simulink library "tqr"  (R2021b)
settings: Solver=VariableStepAuto  StartTime=0.0  StopTime=10.0  RelTol=1e-3
undefined symbols (not defined in the file or in its folder): ATQR_AltRDCActiveREDUInc_X_pct, ATQR_AltRDCActiveREDUInc_Y_enum, ATQR_AltRDCActiveREDUTs_X_pct, ATQR_AltRDCActiveREDUTs_Y_enum, ATQR_CreepREDUTqIncSR_X_rpm, ATQR_CreepREDUTqIncSR_Y_Nm, ATQR_CreepREDUTs_X_rpm, ATQR_CreepREDUTs_Y_Nm, ATQR_EcoTqRrIncGain_X_Nm, ATQR_EcoTqRrIncGain_Y_pct, ATQR_EL1REDUTqDecSR_Y_Nm, ATQR_EL1REDUTqIncSR_X_rpm, ATQR_EL1REDUTqIncSR_Y_pct, ATQR_EL1REDUTs_X_rpm, ATQR_EL1REDUTs_Y_Nm, ATQR_NL1REDUTqDecSR_Y_Nm, ATQR_NL1REDUTqIncSR_X_rpm, ATQR_NL1REDUTqIncSR_Y_pct, ATQR_NL1REDUTs_X_rpm, ATQR_NL1REDUTs_Y_Nm, ATQR_NormalTqRrIncGain_X_Nm, ATQR_NormalTqRrIncGain_Y_pct, ATQR_REDUTIPOutTs_X_rpm, ATQR_RrNegRateLimitIncN_X_rpm, ATQR_RrNegRateLimitIncN_Y_Nm, ATQR_RrPosRateLimitIncN_X_rpm, ATQR_RrPosRateLimitIncN_Y_Nm, ATQR_RTqZeroTransUpBoundN_X_rpm, ATQR_SL1REDUTqDecSR_Y_Nm, ATQR_SL1REDUTqIncSR_X_rpm, ATQR_SL1REDUTqIncSR_Y_pct, ATQR_SL1REDUTs_X_rpm, ATQR_SL1REDUTs_Y_Nm, ATQR_SportTqRrIncGain_X_Nm, ATQR_SportTqRrIncGain_Y_pct, ENUM_CANRDCACTSTA_EXITIMMEDIATELY, ENUM_DRIVEMODE_ECO, ENUM_DRIVEMODE_NRM, ENUM_DRIVEMODE_SPORT, ENUM_GEARACTUALPOSN_R, ENUM_RDCACTSTA_NOREQUEST, ENUM_TQZEROTRANS_NEGATIVE, ENUM_TQZEROTRANS_NOZEROTRANS, ENUM_TQZEROTRANS_POSITIVE, FALSE, KTQD_FrTMTotalGearRatio_gain, KTQD_RrTMTotalGearRatio_gain, KTQR_ARegenLatchEnTq_Nm, KTQR_DriveModeChangeTq_Nm, KTQR_DriveModeCMDTqDev_Nm, KTQR_FinalFEDUTrqLowLim_Nm, KTQR_FinalFEDUTrqUpLim_Nm, KTQR_FinalREDUTrqLowLim_Nm, KTQR_FinalREDUTrqUpLim_Nm, KTQR_FrTMGearEff_c, KTQR_GearEnChangeTq_Nm, KTQR_PreLoadTs_c, KTQR_RrTMGearEff_c, KTQR_TIPOutTsAPS_pct, KTQR_TIPOutTsSpd_kph ... (+44)
libraries: hcu_lib x7, simulink x6
(part 3 of 3)

== system tqr/TQR/Determine Torque Request/TorqueArbitrament/TorqueSmooth/Rear wheel rate limit determination/VTQR_SPORTREDURateLimitInc_Nm ==
  VDHP_ActAPSPosn_pct : Inport
  VTQD_TqTargetShaftSpd_rpm : Inport  Port=2
  VTQD_RegenMode_enum : Inport  Port=3
  VTQR_REDUWhlTqReqSmoothDelay_Nm : Inport  Port=4
  Action Port : ActionPort
  MTQR_SL1REDUTqIncSR_Z_Nm : Lookup_n-D  BreakpointsForDimension1=ATQR_SL1REDUTqIncSR_Y_pct  BreakpointsForDimension2=ATQR_SL1REDUTqIncSR_X_rpm  Table=MTQR_SL1REDUTqIncSR_Z_Nm  ExtrapMethod=Clip  InternalRulePriority=Speed  RndMeth=Simplest  InputSameDT=on
      settings: InputPortMap=u0,u1
  MTQR_SportTqRrIncGain_Z_c : Lookup_n-D  BreakpointsForDimension1=ATQR_SportTqRrIncGain_Y_pct  BreakpointsForDimension2=ATQR_SportTqRrIncGain_X_Nm  Table=MTQR_SportTqRrIncGain_Z_c  ExtrapMethod=Clip  InternalRulePriority=Speed  RndMeth=Simplest  InputSameDT=on
      settings: InputPortMap=u0,u1
  Product : Product
  Terminator : Terminator
  VTQR_SPORTREDURateLimitInc_Nm : Outport
  wires:
  VDHP_ActAPSPosn_pct/1 -> [VDHP_ActAPSPosn_pct]
  VTQD_TqTargetShaftSpd_rpm/1 -> [VTQD_TqTargetShaftSpd_rpm]
  VTQD_RegenMode_enum/1 -> Terminator/1
  [VTQR_REDUWhlTqReqSmoothDelay_Nm] -> MTQR_SportTqRrIncGain_Z_c/2
  [VDHP_ActAPSPosn_pct] -> MTQR_SportTqRrIncGain_Z_c/1
  VTQR_REDUWhlTqReqSmoothDelay_Nm/1 -> [VTQR_REDUWhlTqReqSmoothDelay_Nm]
  MTQR_SportTqRrIncGain_Z_c/1 -> [VTQR_SportTqRrIncGain_c]  "VTQR_SportTqRrIncGain_c"
  MTQR_SL1REDUTqIncSR_Z_Nm/1 -> Product/1
  Product/1 -> VTQR_SPORTREDURateLimitInc_Nm/1  "VTQR_SPORTREDURateLimitInc_Nm"
  [VDHP_ActAPSPosn_pct] -> MTQR_SL1REDUTqIncSR_Z_Nm/1
  [VTQD_TqTargetShaftSpd_rpm] -> MTQR_SL1REDUTqIncSR_Z_Nm/2
  [VTQR_SportTqRrIncGain_c] -> Product/2

== system tqr/TQR/Determine Torque Request/TorqueArbitrament/TorqueSmooth/Rear wheel rate limit determination/Negative Rate limit Determination/VTQR_RrNegRateLimitDecE_Nm ==
  VTQD_TqTargetShaftSpd_rpm : Inport
  VTQR_REDUWhlTqReqSmoothDelay_Nm : Inport  Port=2
  Action Port : ActionPort
  MTQR_RrNegRateLimitDecE_Z_Nm : Lookup_n-D  BreakpointsForDimension1=ATQR_RrNegRateLimitIncN_Y_Nm  BreakpointsForDimension2=ATQR_RrNegRateLimitIncN_X_rpm  Table=MTQR_RrNegRateLimitDecE_Z_Nm  ExtrapMethod=Clip  UseLastTableValue=on  InternalRulePriority=Speed  RndMeth=Simplest  InputSameDT=on
      settings: InputPortMap=u0,u1
  VTQR_RrNegRateLimitDecE_Nm : Outport
  wires:
  MTQR_RrNegRateLimitDecE_Z_Nm/1 -> VTQR_RrNegRateLimitDecE_Nm/1  "VTQR_RrNegRateLimitDecE_Nm"
  VTQR_REDUWhlTqReqSmoothDelay_Nm/1 -> MTQR_RrNegRateLimitDecE_Z_Nm/1
  VTQD_TqTargetShaftSpd_rpm/1 -> MTQR_RrNegRateLimitDecE_Z_Nm/2

== system tqr/TQR/Determine Torque Request/TorqueArbitrament/TorqueSmooth/Rear wheel rate limit determination/Negative Rate limit Determination/VTQR_RrNegRateLimitDecN_Nm ==
  VTQD_TqTargetShaftSpd_rpm : Inport
  VTQR_REDUWhlTqReqSmoothDelay_Nm : Inport  Port=2
  Action Port : ActionPort
  MTQR_RrNegRateLimitDecN_Z_Nm : Lookup_n-D  BreakpointsForDimension1=ATQR_RrNegRateLimitIncN_Y_Nm  BreakpointsForDimension2=ATQR_RrNegRateLimitIncN_X_rpm  Table=MTQR_RrNegRateLimitDecN_Z_Nm  ExtrapMethod=Clip  UseLastTableValue=on  InternalRulePriority=Speed  RndMeth=Simplest  InputSameDT=on
      settings: InputPortMap=u0,u1
  VTQR_RrNegRateLimitDecN_Nm : Outport
  wires:
  MTQR_RrNegRateLimitDecN_Z_Nm/1 -> VTQR_RrNegRateLimitDecN_Nm/1  "VTQR_RrNegRateLimitDecN_Nm"
  VTQR_REDUWhlTqReqSmoothDelay_Nm/1 -> MTQR_RrNegRateLimitDecN_Z_Nm/1
  VTQD_TqTargetShaftSpd_rpm/1 -> MTQR_RrNegRateLimitDecN_Z_Nm/2

== system tqr/TQR/Determine Torque Request/TorqueArbitrament/TorqueSmooth/Rear wheel rate limit determination/Negative Rate limit Determination/VTQR_RrNegRateLimitDecS_Nm ==
  VTQD_TqTargetShaftSpd_rpm : Inport
  VTQR_REDUWhlTqReqSmoothDelay_Nm : Inport  Port=2
  Action Port : ActionPort
  MTQR_RrNegRateLimitDecE_Z_Nm : Lookup_n-D  BreakpointsForDimension1=ATQR_RrNegRateLimitIncN_Y_Nm  BreakpointsForDimension2=ATQR_RrNegRateLimitIncN_X_rpm  Table=MTQR_RrNegRateLimitDecS_Z_Nm  ExtrapMethod=Clip  UseLastTableValue=on  InternalRulePriority=Speed  RndMeth=Simplest  InputSameDT=on
      settings: InputPortMap=u0,u1
  VTQR_RrNegRateLimitDecS_Nm : Outport
  wires:
  MTQR_RrNegRateLimitDecE_Z_Nm/1 -> VTQR_RrNegRateLimitDecS_Nm/1  "VTQR_RrNegRateLimitDecS_Nm"
  VTQD_TqTargetShaftSpd_rpm/1 -> MTQR_RrNegRateLimitDecE_Z_Nm/2
  VTQR_REDUWhlTqReqSmoothDelay_Nm/1 -> MTQR_RrNegRateLimitDecE_Z_Nm/1

== system tqr/TQR/Determine Torque Request/TorqueArbitrament/TorqueSmooth/Rear wheel rate limit determination/Negative Rate limit Determination/VTQR_RrNegRateLimitIncE_Nm ==
  VTQD_TqTargetShaftSpd_rpm : Inport
  VTQR_REDUWhlTqReqSmoothDelay_Nm : Inport  Port=2
  Action Port : ActionPort
  MTQR_RrNegRateLimitIncE_Z_Nm : Lookup_n-D  BreakpointsForDimension1=ATQR_RrNegRateLimitIncN_Y_Nm  BreakpointsForDimension2=ATQR_RrNegRateLimitIncN_X_rpm  Table=MTQR_RrNegRateLimitIncE_Z_Nm  ExtrapMethod=Clip  UseLastTableValue=on  InternalRulePriority=Speed  RndMeth=Simplest  InputSameDT=on
      settings: InputPortMap=u0,u1
  VTQR_RrNegRateLimitIncE_Nm : Outport
  wires:
  MTQR_RrNegRateLimitIncE_Z_Nm/1 -> VTQR_RrNegRateLimitIncE_Nm/1  "VTQR_RrNegRateLimitIncE_Nm"
  VTQR_REDUWhlTqReqSmoothDelay_Nm/1 -> MTQR_RrNegRateLimitIncE_Z_Nm/1
  VTQD_TqTargetShaftSpd_rpm/1 -> MTQR_RrNegRateLimitIncE_Z_Nm/2

== system tqr/TQR/Determine Torque Request/TorqueArbitrament/TorqueSmooth/Rear wheel rate limit determination/Negative Rate limit Determination/VTQR_RrNegRateLimitIncN_Nm ==
  VTQD_TqTargetShaftSpd_rpm : Inport
  VTQR_REDUWhlTqReqSmoothDelay_Nm : Inport  Port=2
  Action Port : ActionPort
  MTQR_RrNegRateLimitIncN_Z_Nm : Lookup_n-D  BreakpointsForDimension1=ATQR_RrNegRateLimitIncN_Y_Nm  BreakpointsForDimension2=ATQR_RrNegRateLimitIncN_X_rpm  Table=MTQR_RrNegRateLimitIncN_Z_Nm  ExtrapMethod=Clip  UseLastTableValue=on  InternalRulePriority=Speed  RndMeth=Simplest  InputSameDT=on
      settings: InputPortMap=u0,u1
  VTQR_RrNegRateLimitIncN_Nm : Outport
  wires:
  MTQR_RrNegRateLimitIncN_Z_Nm/1 -> VTQR_RrNegRateLimitIncN_Nm/1  "VTQR_RrNegRateLimitIncN_Nm"
  VTQR_REDUWhlTqReqSmoothDelay_Nm/1 -> MTQR_RrNegRateLimitIncN_Z_Nm/1
  VTQD_TqTargetShaftSpd_rpm/1 -> MTQR_RrNegRateLimitIncN_Z_Nm/2

== system tqr/TQR/Determine Torque Request/TorqueArbitrament/TorqueSmooth/Rear wheel rate limit determination/Negative Rate limit Determination/VTQR_RrNegRateLimitIncS_Nm ==
  VTQD_TqTargetShaftSpd_rpm : Inport
  VTQR_REDUWhlTqReqSmoothDelay_Nm : Inport  Port=2
  Action Port : ActionPort
  MTQR_RrNegRateLimitIncS_Z_Nm : Lookup_n-D  BreakpointsForDimension1=ATQR_RrNegRateLimitIncN_Y_Nm  BreakpointsForDimension2=ATQR_RrNegRateLimitIncN_X_rpm  Table=MTQR_RrNegRateLimitIncS_Z_Nm  ExtrapMethod=Clip  UseLastTableValue=on  InternalRulePriority=Speed  RndMeth=Simplest  InputSameDT=on
      settings: InputPortMap=u0,u1
  VTQR_RrNegRateLimitIncS_Nm : Outport
  wires:
  MTQR_RrNegRateLimitIncS_Z_Nm/1 -> VTQR_RrNegRateLimitIncS_Nm/1  "VTQR_RrNegRateLimitIncS_Nm"
  VTQD_TqTargetShaftSpd_rpm/1 -> MTQR_RrNegRateLimitIncS_Z_Nm/2
  VTQR_REDUWhlTqReqSmoothDelay_Nm/1 -> MTQR_RrNegRateLimitIncS_Z_Nm/1

== system tqr/TQR/Determine Torque Request/TorqueArbitrament/TorqueSmooth/Rear wheel rate limit determination/Positive Rate limit Determination/VTQR_RrPosRateLimitDecE_Nm ==
  VTQD_TqTargetShaftSpd_rpm : Inport
  VTQR_REDUWhlTqReqSmoothDelay_Nm : Inport  Port=2
  Action Port : ActionPort
  MTQR_RrPosRateLimitDecE_Z_Nm : Lookup_n-D  BreakpointsForDimension1=ATQR_RrPosRateLimitIncN_Y_Nm  BreakpointsForDimension2=ATQR_RrPosRateLimitIncN_X_rpm  Table=MTQR_RrPosRateLimitDecE_Z_Nm  ExtrapMethod=Clip  UseLastTableValue=on  InternalRulePriority=Speed  RndMeth=Simplest  InputSameDT=on
      settings: InputPortMap=u0,u1
  VTQR_RrPosRateLimitDecE_Nm : Outport
  wires:
  VTQD_TqTargetShaftSpd_rpm/1 -> MTQR_RrPosRateLimitDecE_Z_Nm/2
  VTQR_REDUWhlTqReqSmoothDelay_Nm/1 -> MTQR_RrPosRateLimitDecE_Z_Nm/1
  MTQR_RrPosRateLimitDecE_Z_Nm/1 -> VTQR_RrPosRateLimitDecE_Nm/1  "VTQR_RrPosRateLimitDecE_Nm"

== system tqr/TQR/Determine Torque Request/TorqueArbitrament/TorqueSmooth/Rear wheel rate limit determination/Positive Rate limit Determination/VTQR_RrPosRateLimitDecN_Nm ==
  VTQD_TqTargetShaftSpd_rpm : Inport
  VTQR_REDUWhlTqReqSmoothDelay_Nm : Inport  Port=2
  Action Port : ActionPort
  MTQR_RrPosRateLimitDecN_Z_Nm : Lookup_n-D  BreakpointsForDimension1=ATQR_RrPosRateLimitIncN_Y_Nm  BreakpointsForDimension2=ATQR_RrPosRateLimitIncN_X_rpm  Table=MTQR_RrPosRateLimitDecN_Z_Nm  ExtrapMethod=Clip  UseLastTableValue=on  InternalRulePriority=Speed  RndMeth=Simplest  InputSameDT=on
      settings: InputPortMap=u0,u1
  VTQR_RrPosRateLimitDecN_Nm : Outport
  wires:
  VTQD_TqTargetShaftSpd_rpm/1 -> MTQR_RrPosRateLimitDecN_Z_Nm/2
  VTQR_REDUWhlTqReqSmoothDelay_Nm/1 -> MTQR_RrPosRateLimitDecN_Z_Nm/1
  MTQR_RrPosRateLimitDecN_Z_Nm/1 -> VTQR_RrPosRateLimitDecN_Nm/1  "VTQR_RrPosRateLimitDecN_Nm"

== system tqr/TQR/Determine Torque Request/TorqueArbitrament/TorqueSmooth/Rear wheel rate limit determination/Positive Rate limit Determination/VTQR_RrPosRateLimitDecS_Nm ==
  VTQD_TqTargetShaftSpd_rpm : Inport
  VTQR_REDUWhlTqReqSmoothDelay_Nm : Inport  Port=2
  Action Port : ActionPort
  MTQR_RrPosRateLimitDecE_Z_Nm : Lookup_n-D  BreakpointsForDimension1=ATQR_RrPosRateLimitIncN_Y_Nm  BreakpointsForDimension2=ATQR_RrPosRateLimitIncN_X_rpm  Table=MTQR_RrPosRateLimitDecS_Z_Nm  ExtrapMethod=Clip  UseLastTableValue=on  InternalRulePriority=Speed  RndMeth=Simplest  InputSameDT=on
      settings: InputPortMap=u0,u1
  VTQR_RrPosRateLimitDecS_Nm : Outport
  wires:
  VTQR_REDUWhlTqReqSmoothDelay_Nm/1 -> MTQR_RrPosRateLimitDecE_Z_Nm/1
  VTQD_TqTargetShaftSpd_rpm/1 -> MTQR_RrPosRateLimitDecE_Z_Nm/2
  MTQR_RrPosRateLimitDecE_Z_Nm/1 -> VTQR_RrPosRateLimitDecS_Nm/1  "VTQR_RrPosRateLimitDecS_Nm"

== system tqr/TQR/Determine Torque Request/TorqueArbitrament/TorqueSmooth/Rear wheel rate limit determination/Positive Rate limit Determination/VTQR_RrPosRateLimitIncE_Nm ==
  VTQD_TqTargetShaftSpd_rpm : Inport
  VTQR_REDUWhlTqReqSmoothDelay_Nm : Inport  Port=2
  Action Port : ActionPort
  MTQR_RrPosRateLimitIncE_Z_Nm : Lookup_n-D  BreakpointsForDimension1=ATQR_RrPosRateLimitIncN_Y_Nm  BreakpointsForDimension2=ATQR_RrPosRateLimitIncN_X_rpm  Table=MTQR_RrPosRateLimitIncE_Z_Nm  ExtrapMethod=Clip  UseLastTableValue=on  InternalRulePriority=Speed  RndMeth=Simplest  InputSameDT=on
      settings: InputPortMap=u0,u1
  VTQR_RrPosRateLimitIncE_Nm : Outport
  wires:
  VTQD_TqTargetShaftSpd_rpm/1 -> MTQR_RrPosRateLimitIncE_Z_Nm/2
  VTQR_REDUWhlTqReqSmoothDelay_Nm/1 -> MTQR_RrPosRateLimitIncE_Z_Nm/1
  MTQR_RrPosRateLimitIncE_Z_Nm/1 -> VTQR_RrPosRateLimitIncE_Nm/1  "VTQR_RrPosRateLimitIncE_Nm"

== system tqr/TQR/Determine Torque Request/TorqueArbitrament/TorqueSmooth/Rear wheel rate limit determination/Positive Rate limit Determination/VTQR_RrPosRateLimitIncN_Nm ==
  VTQD_TqTargetShaftSpd_rpm : Inport
  VTQR_REDUWhlTqReqSmoothDelay_Nm : Inport  Port=2
  Action Port : ActionPort
  MTQR_RrPosRateLimitIncN_Z_Nm : Lookup_n-D  BreakpointsForDimension1=ATQR_RrPosRateLimitIncN_Y_Nm  BreakpointsForDimension2=ATQR_RrPosRateLimitIncN_X_rpm  Table=MTQR_RrPosRateLimitIncN_Z_Nm  ExtrapMethod=Clip  UseLastTableValue=on  InternalRulePriority=Speed  RndMeth=Simplest  InputSameDT=on
      settings: InputPortMap=u0,u1
  VTQR_RrPosRateLimitIncN_Nm : Outport
  wires:
  VTQD_TqTargetShaftSpd_rpm/1 -> MTQR_RrPosRateLimitIncN_Z_Nm/2
  VTQR_REDUWhlTqReqSmoothDelay_Nm/1 -> MTQR_RrPosRateLimitIncN_Z_Nm/1
  MTQR_RrPosRateLimitIncN_Z_Nm/1 -> VTQR_RrPosRateLimitIncN_Nm/1  "VTQR_RrPosRateLimitIncN_Nm"

== system tqr/TQR/Determine Torque Request/TorqueArbitrament/TorqueSmooth/Rear wheel rate limit determination/Positive Rate limit Determination/VTQR_RrPosRateLimitIncS_Nm ==
  VTQD_TqTargetShaftSpd_rpm : Inport
  VTQR_REDUWhlTqReqSmoothDelay_Nm : Inport  Port=2
  Action Port : ActionPort
  MTQR_RrPosRateLimitIncS_Z_Nm : Lookup_n-D  BreakpointsForDimension1=ATQR_RrPosRateLimitIncN_Y_Nm  BreakpointsForDimension2=ATQR_RrPosRateLimitIncN_X_rpm  Table=MTQR_RrPosRateLimitIncS_Z_Nm  ExtrapMethod=Clip  UseLastTableValue=on  InternalRulePriority=Speed  RndMeth=Simplest  InputSameDT=on
      settings: InputPortMap=u0,u1
  VTQR_RrPosRateLimitIncS_Nm : Outport
  wires:
  VTQR_REDUWhlTqReqSmoothDelay_Nm/1 -> MTQR_RrPosRateLimitIncS_Z_Nm/1
  VTQD_TqTargetShaftSpd_rpm/1 -> MTQR_RrPosRateLimitIncS_Z_Nm/2
  MTQR_RrPosRateLimitIncS_Z_Nm/1 -> VTQR_RrPosRateLimitIncS_Nm/1  "VTQR_RrPosRateLimitIncS_Nm"
